simulink model "Telecontrol"  (R2024b)
settings: Solver=ode5  StartTime=0.0  StopTime=inf  FixedStep=1/600  RelTol=1e-3
undefined symbols (not defined in the file): Low
libraries: arduinolib x42, dspswit3 x12, etargetslib x10, simulink x6, canmsglib x6, svdutilitieslib x1
settings Model: SimulationMode=external  Creator=alexx  LastModifiedBy=Marwa
settings SolverCC: AutoInsertRateTranBlk=on
settings OptimizationCC: EnhancedBackFolding=on  PassReuseOutputArgsAs=Individual arguments  ZeroExternalMemoryAtStartup=off  ZeroInternalMemoryAtStartup=off  MaxStackSize=64  OptimizeBlockOrder=speed  DifferentSizesBufferReuse=on  OptimizationCustomize=off  EfficientTunableParamExpr=on
settings DebuggingCC: ParameterTunabilityLossMsg=error
settings HardwareCC: ProdBitPerPointer=32  ProdBitPerSizeT=32  ProdBitPerPtrDiffT=32  ProdLargestAtomicInteger=Long  ProdLargestAtomicFloat=Double  ProdWordSize=32  ProdHWDeviceType=ARM Compatible->ARM Cortex  UseEmbeddedCoderFeatures=off
settings SFSimCC: MATLABDynamicMemAlloc=off
settings RTWCC: Description=Embedded Coder  SystemTargetFile=ert.tlc  HardwareBoard=Arduino MKR WiFi 1010  TemplateMakefile=ert_default_tmf  Toolchain=Arduino ARM  BuildConfiguration=Faster Runs  GPUComputeCapability=3.5
settings CodeAppCC: ForceParamTrailComments=on  IgnoreCustomStorageClasses=off  OperatorAnnotations=on  SimulinkDataObjDesc=on  SFDataObjDesc=on  InsertBlockDesc=on
settings ERTTargetCC: SupportContinuousTime=on  SupportNonInlinedSFcns=on  SupportVariableSizeSignals=on  ExtModeTransport=3  ExtModeStaticAlloc=on  ExtModeAutomaticAllocSize=off  ExtModeStaticAllocSize=8192  ExtModeMexFile=ext_xcp  ExtModeIntrfLevel=Level2 - Open  InlinedParameterPlacement=Hierarchical  DynamicArrayContainerType=coder::array

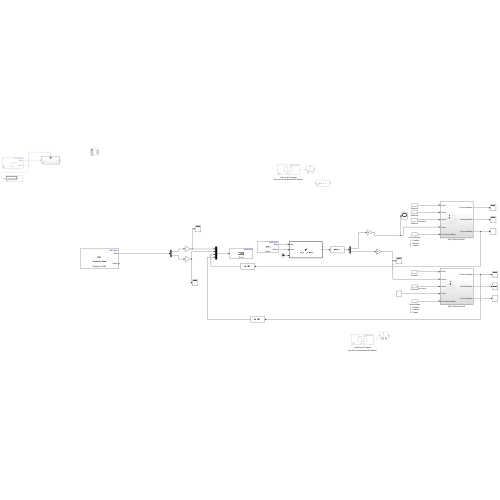
[thumbnail: Simulink's stored preview of the top-level diagram]
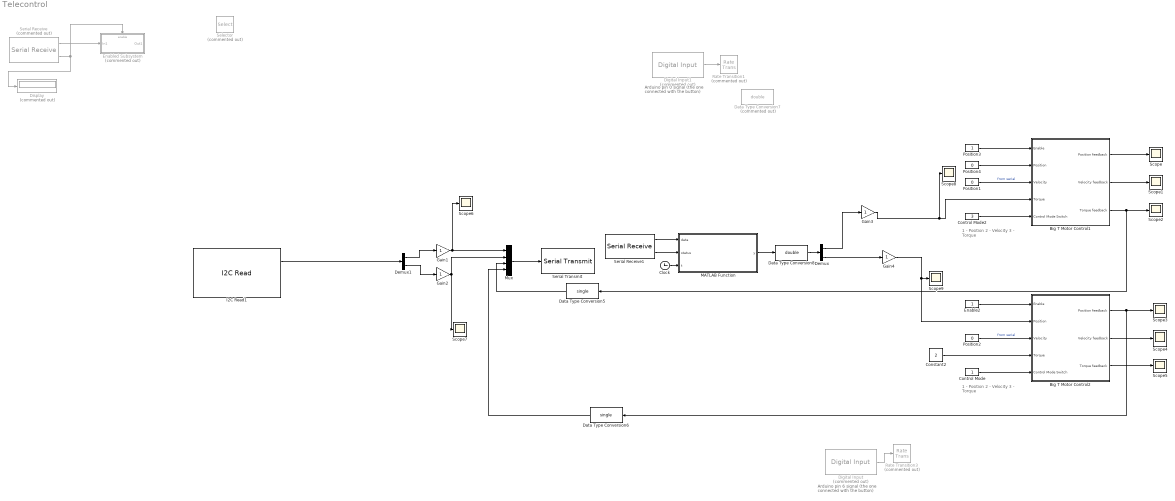
== system Telecontrol ==
  note: 1 - Position
      | 2 - Velocity
      | 3 - Torque
  note: Arduino pin 6 signal
      | (the one connected with the button)
  note: Arduino pin 0 signal
      | (the one connected with the button)
  note: 1 - Position
      | 2 - Velocity
      | 3 - Torque
  Big T Motor Control1 : Subsystem
  Big T Motor Control2 : Subsystem
  Clock : Clock
  Constant2 : Constant  Value=2
  Control Mode : Constant
  Control Mode2 : Constant  Value=3
  Data Type Conversion5 : DataTypeConversion  OutDataTypeStr=single  SaturateOnIntegerOverflow=off  RndMeth=Floor
  Data Type Conversion6 : DataTypeConversion  OutDataTypeStr=single  SaturateOnIntegerOverflow=off  RndMeth=Floor
  Data Type Conversion7 : DataTypeConversion  Commented=on  OutDataTypeStr=double  SaturateOnIntegerOverflow=off  RndMeth=Floor
  Data Type Conversion8 : DataTypeConversion  OutDataTypeStr=double  SaturateOnIntegerOverflow=off  RndMeth=Floor
  Demux : Demux  Outputs=2
  Demux1 : Demux  Outputs=2
  Digital Input : arduinolib/Digital Input  Commented=on  pinNumber=6  mode=Default  Direction=input  SampleTime=0.01  blockPlatform=arduino
      settings: SourceProductName=Common
  Digital Input1 : arduinolib/Digital Input  Commented=on  pinNumber=0  mode=Default  Direction=input  SampleTime=0.01  blockPlatform=arduino
      settings: SourceProductName=Common
  Display : Display  Commented=on
  Enable2 : Constant
  Enabled Subsystem : Subsystem  Commented=on  TreatAsAtomicUnit=on
  Gain{1..4} (4 alike) : Gain
  I2C Read1 : arduinolib/I2C Read  I2CModule=0  Mode=Master  SlaveAddress=45  SlaveByteOrder=LittleEndian  Direction=Receiver  RegisterAddressMode=off  RegisterAddress=0  SlaveDataType=single  DataLength=2  NoAck=off  RepeatedStart=off  OutputStatus=on  blockPlatform=ARDUINO  SampleTime=1/300
      settings: SourceProductName=Common
  MATLAB Function : MATLAB Function  TreatAsAtomicUnit=on
  Mux : Mux
  Position1 : Constant  Value=0
  Position2 : Constant  Value=0
  Position3 : Constant
  Position4 : Constant  Value=0
  Rate Transition1 : RateTransition  Commented=on  OutPortSampleTime=0.01
  Rate Transition3 : RateTransition  Commented=on  OutPortSampleTime=0.01
  Scope{,1..9} (10 alike) : Scope
  Selector : Selector  Commented=on  InputPortWidth=4  IndexOptions=Index vector (dialog)  Indices=[2 3]  OutputSizes=1
  Serial Receive : arduinolib/Serial Receive  Commented=on  portNumber=1  DataType=uint8  blockPlatform=ARDUINO  TimeOut=100  MaxDataLength=8  isARMArch=off  DataLengthOption=Length via dialog  Datalength=8  Header=[170.0]  Terminator=[187.0]  SampleTime=0.001  ShowOutStatus=on
      settings: SourceProductName=Common
  Serial Receive1 : arduinolib/Serial Receive  portNumber=0  DataType=single  blockPlatform=ARDUINO  TimeOut=0  MaxDataLength=10  isARMArch=off  DataLengthOption=Length via dialog  Datalength=2  Header=[170 85]  Terminator=[]  SampleTime=1/300  ShowOutStatus=on
      settings: SourceProductName=Common
  Serial Transmit : arduinolib/Serial Transmit  portNumber=0  sendmode=write  sendformat=Decimal  floatprecision=2  header=[170 85]  terminator=[]  blockPlatform=ARDUINO
      settings: SourceProductName=Common
  wires:
  Control Mode2/1 -> Big T Motor Control1/5(Control Mode Switch)
  Digital Input/1 -> Rate Transition3/1
  Position4/1 -> Big T Motor Control1/2(Position)
  Control Mode/1 -> Big T Motor Control2/5(Control Mode Switch)
  Big T Motor Control1/1(Position feedback) -> Scope/1
  Big T Motor Control1/2(Velocity feedback) -> Scope1/1
  Big T Motor Control1/3(Torque feedback) -> Data Type Conversion5/1, Scope2/1
  Big T Motor Control2/1(Position feedback) -> Data Type Conversion6/1, Scope3/1
  Big T Motor Control2/2(Velocity feedback) -> Scope4/1
  Big T Motor Control2/3(Torque feedback) -> Scope5/1
  Digital Input1/1 -> Rate Transition1/1
  Position1/1 -> Big T Motor Control1/3(Velocity)  "from serial"
  Constant2/1 -> Big T Motor Control2/4(Torque)
  Position2/1 -> Big T Motor Control2/3(Velocity)  "from serial"
  Serial Receive/2 -> Display/1, Enabled Subsystem/Enable
  Serial Receive/1 -> Enabled Subsystem/1(In1)
  Position3/1 -> Big T Motor Control1/1(Enable)
  Enable2/1 -> Big T Motor Control2/1(Enable)
  Serial Receive1/2 -> MATLAB Function/2(status)
  Mux/1 -> Serial Transmit/1
  Gain1/1 -> Mux/1, Scope6/1
  Gain2/1 -> Scope7/1, Mux/2
  Gain3/1 -> Scope8/1, Big T Motor Control1/4(Torque)
  Gain4/1 -> Big T Motor Control2/2(Position), Scope9/1
  Data Type Conversion8/1 -> Demux/1
  Demux/2 -> Gain4/1
  Demux/1 -> Gain3/1
  Data Type Conversion5/1 -> Mux/3
  Data Type Conversion6/1 -> Mux/4
  Serial Receive1/1 -> MATLAB Function/1(data)
  MATLAB Function/1(y) -> Data Type Conversion8/1
  Clock/1 -> MATLAB Function/3(t)
  I2C Read1/1 -> Demux1/1
  Demux1/1 -> Gain1/1
  Demux1/2 -> Gain2/1

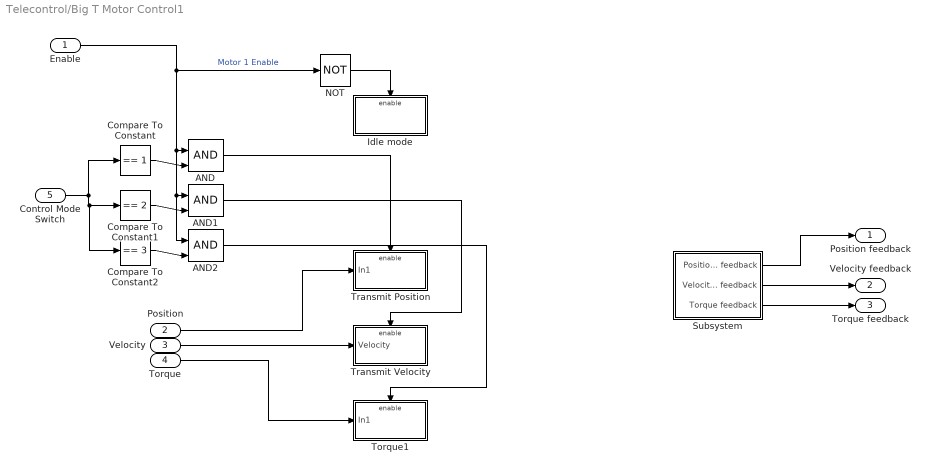
== system Telecontrol/Big T Motor Control1 ==
  Enable : Inport
  Position : Inport  Port=2  Unit=rad
  Velocity : Inport  Port=3  Unit=rad/s
  Torque : Inport  Port=4  Unit=N*m
  Control Mode Switch : Inport  Port=5
  AND : Logic  IconShape=distinctive  AllPortsSameDT=off  OutDataTypeStr=boolean
  AND1 : Logic  IconShape=distinctive  AllPortsSameDT=off  OutDataTypeStr=boolean
  AND2 : Logic  IconShape=distinctive  AllPortsSameDT=off  OutDataTypeStr=boolean
  Compare To Constant : simulink/Logic and Bit Operations/Compare To Constant  relop===  const=1  OutDataTypeStr=boolean
  Compare To Constant1 : simulink/Logic and Bit Operations/Compare To Constant  relop===  const=2  OutDataTypeStr=boolean
  Compare To Constant2 : simulink/Logic and Bit Operations/Compare To Constant  relop===  const=3  OutDataTypeStr=boolean
  Idle mode : Subsystem  TreatAsAtomicUnit=on
  NOT : Logic  Operator=NOT  AllPortsSameDT=off  OutDataTypeStr=boolean
  Subsystem : Subsystem
  Torque1 : Subsystem  TreatAsAtomicUnit=on
  Transmit Position : Subsystem  TreatAsAtomicUnit=on
  Transmit Velocity : Subsystem  TreatAsAtomicUnit=on
  Position feedback : Outport
  Velocity feedback : Outport  Port=2
  Torque feedback : Outport  Port=3
  wires:
  Position/1 -> Transmit Position/1(In1)
  Torque/1 -> Torque1/1(In1)
  Enable/1 -> AND2/1, AND1/1, AND/1, NOT/1  "Motor 1 Enable"
  NOT/1 -> Idle mode/Enable
  Control Mode Switch/1 -> Compare To Constant2/1, Compare To Constant1/1, Compare To Constant/1
  Velocity/1 -> Transmit Velocity/1(Velocity)
  Compare To Constant/1 -> AND/2
  AND/1 -> Transmit Position/Enable
  Compare To Constant1/1 -> AND1/2
  AND1/1 -> Transmit Velocity/Enable
  Compare To Constant2/1 -> AND2/2
  AND2/1 -> Torque1/Enable
  Subsystem/2(Velocity feedback) -> Velocity feedback/1
  Subsystem/1(Position feedback) -> Position feedback/1
  Subsystem/3(Torque feedback) -> Torque feedback/1

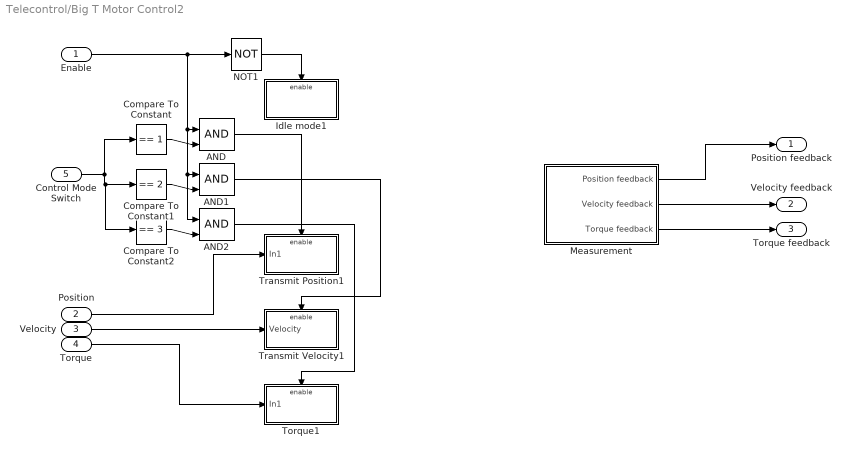
== system Telecontrol/Big T Motor Control2 ==
  Enable : Inport
  Position : Inport  Port=2  Unit=rad
  Velocity : Inport  Port=3  Unit=rad/s
  Torque : Inport  Port=4  Unit=N*m
  Control Mode Switch : Inport  Port=5
  AND : Logic  IconShape=distinctive  AllPortsSameDT=off  OutDataTypeStr=boolean
  AND1 : Logic  IconShape=distinctive  AllPortsSameDT=off  OutDataTypeStr=boolean
  AND2 : Logic  IconShape=distinctive  AllPortsSameDT=off  OutDataTypeStr=boolean
  Compare To Constant : simulink/Logic and Bit Operations/Compare To Constant  relop===  const=1  OutDataTypeStr=boolean
  Compare To Constant1 : simulink/Logic and Bit Operations/Compare To Constant  relop===  const=2  OutDataTypeStr=boolean
  Compare To Constant2 : simulink/Logic and Bit Operations/Compare To Constant  relop===  const=3  OutDataTypeStr=boolean
  Idle mode1 : Subsystem  TreatAsAtomicUnit=on
  Measurement : Subsystem
  NOT1 : Logic  Operator=NOT  AllPortsSameDT=off  OutDataTypeStr=boolean
  Torque1 : Subsystem  TreatAsAtomicUnit=on
  Transmit Position1 : Subsystem  TreatAsAtomicUnit=on
  Transmit Velocity1 : Subsystem  TreatAsAtomicUnit=on
  Position feedback : Outport
  Velocity feedback : Outport  Port=2
  Torque feedback : Outport  Port=3
  wires:
  Velocity/1 -> Transmit Velocity1/1(Velocity)
  Position/1 -> Transmit Position1/1(In1)
  Torque/1 -> Torque1/1(In1)
  NOT1/1 -> Idle mode1/Enable
  AND2/1 -> Torque1/Enable
  Control Mode Switch/1 -> Compare To Constant2/1, Compare To Constant1/1, Compare To Constant/1
  Compare To Constant1/1 -> AND1/2
  AND1/1 -> Transmit Velocity1/Enable
  Compare To Constant/1 -> AND/2
  Compare To Constant2/1 -> AND2/2
  AND/1 -> Transmit Position1/Enable
  Enable/1 -> NOT1/1, AND/1, AND2/1, AND1/1
  Measurement/1(Position feedback) -> Position feedback/1
  Measurement/2(Velocity feedback) -> Velocity feedback/1
  Measurement/3(Torque feedback) -> Torque feedback/1

== system Telecontrol/Enabled Subsystem ==
  In1 : Inport
  Enable : EnablePort
  Byte Unpack : svdutilitieslib/Byte Unpack  dimensions={[2]}  datatypes={'single'}  byteAlign=1  blockPlatform=arduinoert
  Out1 : Outport
  wires:
  In1/1 -> Byte Unpack/1
  Byte Unpack/1 -> Out1/1

== system Telecontrol/Big T Motor Control1/Idle mode ==
  Enable : EnablePort
  CAN Transmit1 : arduinolib/CAN Transmit  inputDataType=Raw data  BlockingMode_=off  BlockTimeout_=1  outputStatus=off  identifierType=Extended (29-bit identifier)  messageId=2097192  msgLength=0  remoteFrame=off
      settings: SourceProductName=Common

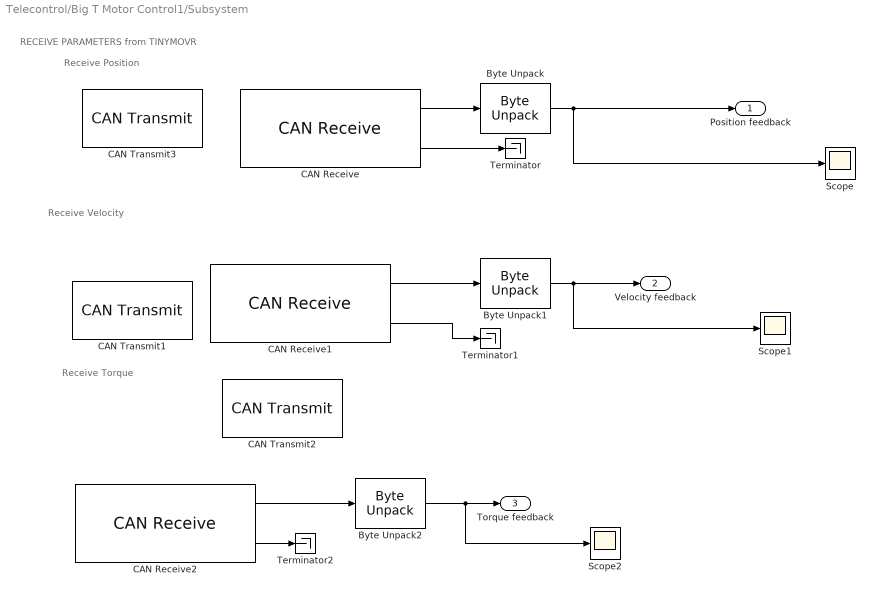
== system Telecontrol/Big T Motor Control1/Subsystem ==
  note: Receive Torque
  note: Receive Velocity
  note: Receive Position
  note: RECEIVE PARAMETERS from TINYMOVR
  Byte Unpack : etargetslib/Byte Unpack  dimensions={[1]}  datatypes={'single'}  byteAlign=1
  Byte Unpack1 : etargetslib/Byte Unpack  dimensions={[1]}  datatypes={'single'}  byteAlign=1
  Byte Unpack2 : etargetslib/Byte Unpack  dimensions={[1]}  datatypes={'single'}  byteAlign=1
  CAN Receive : arduinolib/CAN Receive  outputDataType=Raw data  identifierType=Extended (29-bit identifier)  messageId=2097207  msgLength=4  SampleTime=1/100  outputError=off  outputRemote=off
      settings: SourceProductName=Common
  CAN Receive1 : arduinolib/CAN Receive  outputDataType=Raw data  identifierType=Extended (29-bit identifier)  messageId=2097208  msgLength=4  SampleTime=1/100  outputError=off  outputRemote=off
      settings: SourceProductName=Common
  CAN Receive2 : arduinolib/CAN Receive  outputDataType=Raw data  identifierType=Extended (29-bit identifier)  messageId=2097185  msgLength=4  SampleTime=-1  outputError=off  outputRemote=off
      settings: SourceProductName=Common
  CAN Transmit1 : arduinolib/CAN Transmit  inputDataType=Raw data  BlockingMode_=off  BlockTimeout_=1  outputStatus=off  identifierType=Extended (29-bit identifier)  messageId=2097208  msgLength=0  remoteFrame=on
      settings: SourceProductName=Common
  CAN Transmit2 : arduinolib/CAN Transmit  inputDataType=Raw data  BlockingMode_=off  BlockTimeout_=1  outputStatus=off  identifierType=Extended (29-bit identifier)  messageId=2097185  msgLength=0  remoteFrame=on
      settings: SourceProductName=Common
  CAN Transmit3 : arduinolib/CAN Transmit  inputDataType=Raw data  BlockingMode_=off  BlockTimeout_=1  outputStatus=off  identifierType=Extended (29-bit identifier)  messageId=2097207  msgLength=0  remoteFrame=on
      settings: SourceProductName=Common
  Scope : Scope
  Scope1 : Scope
  Scope2 : Scope
  Terminator : Terminator
  Terminator1 : Terminator
  Terminator2 : Terminator
  Position feedback : Outport
  Velocity feedback : Outport  Port=2
  Torque feedback : Outport  Port=3
  wires:
  CAN Receive1/2 -> Terminator1/1
  Byte Unpack/1 -> Position feedback/1, Scope/1
  CAN Receive/1 -> Byte Unpack/1
  CAN Receive2/1 -> Byte Unpack2/1
  Byte Unpack2/1 -> Torque feedback/1, Scope2/1
  CAN Receive1/1 -> Byte Unpack1/1
  CAN Receive/2 -> Terminator/1
  Byte Unpack1/1 -> Velocity feedback/1, Scope1/1
  CAN Receive2/2 -> Terminator2/1

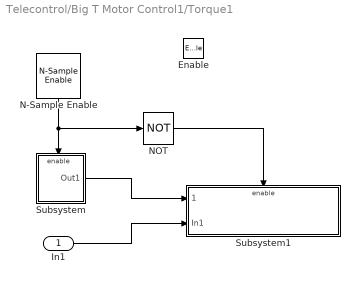
== system Telecontrol/Big T Motor Control1/Torque1 ==
  In1 : Inport
  Enable : EnablePort
  N-Sample Enable : dspswit3/N-Sample Enable  N=5  ActiveLevel=Low (0)  reset=off  TriggerType=Rising edge  Ts=1/100  DataType=Logical
  NOT : Logic  Operator=NOT  IconShape=distinctive  AllPortsSameDT=off  OutDataTypeStr=boolean
  Subsystem : Subsystem
  Subsystem1 : Subsystem
  wires:
  N-Sample Enable/1 -> Subsystem/Enable, NOT/1
  Subsystem/1(Out1) -> Subsystem1/1(" ")
  In1/1 -> Subsystem1/2(In1)
  NOT/1 -> Subsystem1/Enable

== system Telecontrol/Big T Motor Control1/Transmit Position ==
  In1 : Inport
  Enable : EnablePort
  N-Sample Enable : dspswit3/N-Sample Enable  N=5  ActiveLevel=Low (0)  reset=off  TriggerType=Rising edge  Ts=1/100  DataType=Logical
  NOT : Logic  Operator=NOT  IconShape=distinctive  AllPortsSameDT=off  OutDataTypeStr=boolean
  Subsystem : Subsystem
  Subsystem1 : Subsystem
  wires:
  N-Sample Enable/1 -> Subsystem/Enable, NOT/1
  Subsystem/1(Out1) -> Subsystem1/1(" ")
  In1/1 -> Subsystem1/2(In1)
  NOT/1 -> Subsystem1/Enable

== system Telecontrol/Big T Motor Control1/Transmit Velocity ==
  Velocity : Inport
  Enable : EnablePort
  N-Sample Enable : dspswit3/N-Sample Enable  N=5  ActiveLevel=Low (0)  reset=off  TriggerType=Rising edge  Ts=1/100  DataType=Logical
  NOT : Logic  Operator=NOT  IconShape=distinctive  AllPortsSameDT=off  OutDataTypeStr=boolean
  Subsystem : Subsystem
  Subsystem1 : Subsystem
  wires:
  N-Sample Enable/1 -> Subsystem/Enable, NOT/1
  Velocity/1 -> Subsystem1/1(Velocity)
  NOT/1 -> Subsystem1/Enable

== system Telecontrol/Big T Motor Control2/Idle mode1 ==
  Enable : EnablePort
  CAN Transmit1 : arduinolib/CAN Transmit  inputDataType=Raw data  BlockingMode_=off  BlockTimeout_=1  outputStatus=off  identifierType=Extended (29-bit identifier)  messageId=4194344  msgLength=0  remoteFrame=off
      settings: SourceProductName=Common

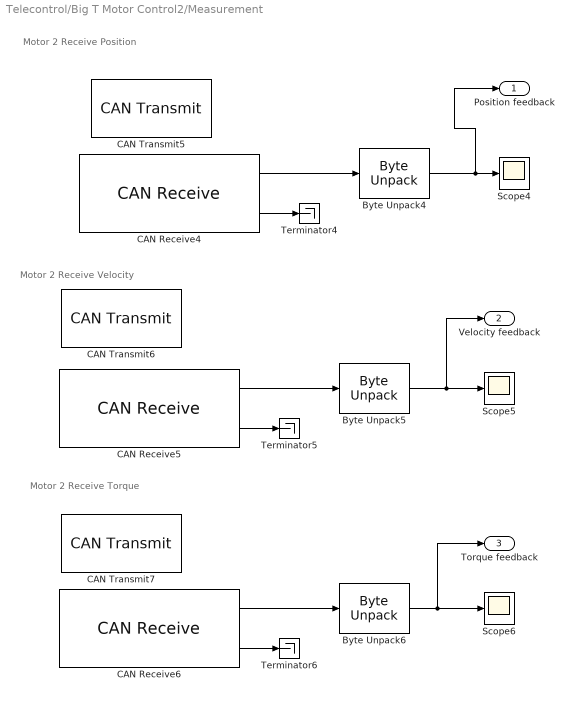
== system Telecontrol/Big T Motor Control2/Measurement ==
  note: Motor 2 Receive Torque
  note: Motor 2 Receive Velocity
  note: Motor 2 Receive Position
  Byte Unpack4 : etargetslib/Byte Unpack  dimensions={[1]}  datatypes={'single'}  byteAlign=1
  Byte Unpack5 : etargetslib/Byte Unpack  dimensions={[1]}  datatypes={'single'}  byteAlign=1
  Byte Unpack6 : etargetslib/Byte Unpack  dimensions={[1]}  datatypes={'single'}  byteAlign=1
  CAN Receive4 : arduinolib/CAN Receive  outputDataType=Raw data  identifierType=Extended (29-bit identifier)  messageId=4194359  msgLength=4  SampleTime=0.01  outputError=off  outputRemote=off
      settings: SourceProductName=Common
  CAN Receive5 : arduinolib/CAN Receive  outputDataType=Raw data  identifierType=Extended (29-bit identifier)  messageId=4194360  msgLength=4  SampleTime=0.01  outputError=off  outputRemote=off
      settings: SourceProductName=Common
  CAN Receive6 : arduinolib/CAN Receive  outputDataType=Raw data  identifierType=Extended (29-bit identifier)  messageId=4194337  msgLength=4  SampleTime=0.01  outputError=off  outputRemote=off
      settings: SourceProductName=Common
  CAN Transmit5 : arduinolib/CAN Transmit  inputDataType=Raw data  BlockingMode_=off  BlockTimeout_=1  outputStatus=off  identifierType=Extended (29-bit identifier)  messageId=4194359  msgLength=0  remoteFrame=on
      settings: SourceProductName=Common
  CAN Transmit6 : arduinolib/CAN Transmit  inputDataType=Raw data  BlockingMode_=off  BlockTimeout_=1  outputStatus=off  identifierType=Extended (29-bit identifier)  messageId=4194360  msgLength=0  remoteFrame=on
      settings: SourceProductName=Common
  CAN Transmit7 : arduinolib/CAN Transmit  inputDataType=Raw data  BlockingMode_=off  BlockTimeout_=1  outputStatus=off  identifierType=Extended (29-bit identifier)  messageId=4194337  msgLength=0  remoteFrame=on
      settings: SourceProductName=Common
  Scope4 : Scope
  Scope5 : Scope
  Scope6 : Scope
  Terminator4 : Terminator
  Terminator5 : Terminator
  Terminator6 : Terminator
  Position feedback : Outport
  Velocity feedback : Outport  Port=2
  Torque feedback : Outport  Port=3
  wires:
  CAN Receive5/1 -> Byte Unpack5/1
  CAN Receive4/1 -> Byte Unpack4/1
  Byte Unpack4/1 -> Position feedback/1, Scope4/1
  CAN Receive6/2 -> Terminator6/1
  CAN Receive6/1 -> Byte Unpack6/1
  Byte Unpack5/1 -> Velocity feedback/1, Scope5/1
  CAN Receive5/2 -> Terminator5/1
  CAN Receive4/2 -> Terminator4/1
  Byte Unpack6/1 -> Torque feedback/1, Scope6/1

== system Telecontrol/Big T Motor Control2/Torque1 ==
  In1 : Inport
  Enable : EnablePort
  N-Sample Enable : dspswit3/N-Sample Enable  N=5  ActiveLevel=Low (0)  reset=off  TriggerType=Rising edge  Ts=1/100  DataType=Logical
  NOT : Logic  Operator=NOT  IconShape=distinctive  AllPortsSameDT=off  OutDataTypeStr=boolean
  Subsystem : Subsystem
  Subsystem1 : Subsystem
  wires:
  N-Sample Enable/1 -> Subsystem/Enable, NOT/1
  Subsystem/1(Out1) -> Subsystem1/1(" ")
  In1/1 -> Subsystem1/2(In1)
  NOT/1 -> Subsystem1/Enable

== system Telecontrol/Big T Motor Control2/Transmit Position1 ==
  In1 : Inport
  Enable : EnablePort
  N-Sample Enable : dspswit3/N-Sample Enable  N=5  ActiveLevel=Low (0)  reset=off  TriggerType=Rising edge  Ts=1/100  DataType=Logical
  NOT : Logic  Operator=NOT  IconShape=distinctive  AllPortsSameDT=off  OutDataTypeStr=boolean
  Subsystem : Subsystem
  Subsystem1 : Subsystem
  wires:
  N-Sample Enable/1 -> Subsystem/Enable, NOT/1
  Subsystem/1(Out1) -> Subsystem1/1(" ")
  In1/1 -> Subsystem1/2(In1)
  NOT/1 -> Subsystem1/Enable

== system Telecontrol/Big T Motor Control2/Transmit Velocity1 ==
  Velocity : Inport
  Enable : EnablePort
  N-Sample Enable : dspswit3/N-Sample Enable  N=5  ActiveLevel=Low (0)  reset=off  TriggerType=Rising edge  Ts=1/100  DataType=Logical
  NOT : Logic  Operator=NOT  IconShape=distinctive  AllPortsSameDT=off  OutDataTypeStr=boolean
  Subsystem : Subsystem
  Subsystem1 : Subsystem
  wires:
  N-Sample Enable/1 -> Subsystem/Enable, NOT/1
  Velocity/1 -> Subsystem1/1(Velocity)
  NOT/1 -> Subsystem1/Enable

== system Telecontrol/Big T Motor Control1/Torque1/Subsystem ==
  Enable : EnablePort
  Byte Unpack : etargetslib/Byte Unpack  dimensions={[1]}  datatypes={'single'}  byteAlign=1
  CAN Receive : arduinolib/CAN Receive  outputDataType=Raw data  identifierType=Extended (29-bit identifier)  messageId=2097185  msgLength=4  SampleTime=1/100  outputError=off  outputRemote=off
      settings: SourceProductName=Common
  CAN Transmit3 : arduinolib/CAN Transmit  inputDataType=Raw data  BlockingMode_=off  BlockTimeout_=1  outputStatus=off  identifierType=Extended (29-bit identifier)  messageId=2097185  msgLength=0  remoteFrame=on
      settings: SourceProductName=Common
  Terminator : Terminator
  Out1 : Outport
  wires:
  CAN Receive/2 -> Terminator/1
  CAN Receive/1 -> Byte Unpack/1
  Byte Unpack/1 -> Out1/1

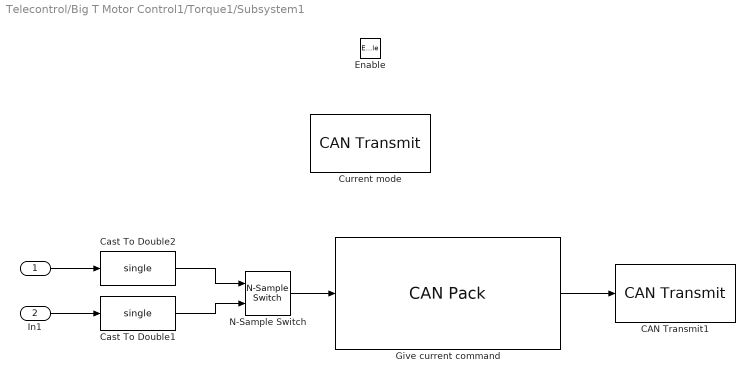
== system Telecontrol/Big T Motor Control1/Torque1/Subsystem1 ==
  " " : Inport
  In1 : Inport  Port=2
  Enable : EnablePort
  CAN Transmit1 : arduinolib/CAN Transmit  inputDataType=CAN Msg  BlockingMode_=off  BlockTimeout_=1  outputStatus=off  identifierType=Extended (29-bit identifier)  messageId=position_setpoint  msgLength=4  remoteFrame=off
      settings: SourceProductName=Common
  Cast To Double1 : DataTypeConversion  OutDataTypeStr=single  SaturateOnIntegerOverflow=off  RndMeth=Floor
  Cast To Double2 : DataTypeConversion  OutDataTypeStr=single  SaturateOnIntegerOverflow=off  RndMeth=Floor
  Current mode : arduinolib/CAN Transmit  inputDataType=Raw data  BlockingMode_=off  BlockTimeout_=1  outputStatus=off  identifierType=Extended (29-bit identifier)  messageId=2097195  msgLength=0  remoteFrame=off
      settings: SourceProductName=Common
  Give current command : canmsglib/CAN Pack  MsgList=(none)  MsgName=CAN Msg  MsgIDType=Extended (29-bit identifier)  MsgIdentifier=2097182  CANIDInput=off  MsgLength=4  Remote=off  ApplyMinMax=off  BusOutput=on  SignalInfo={ 'position', '0', '32', 'LE', 'single', 'Standard', '0', '1', '0', '-Inf', 'Inf' }
      settings: DataFormat=manually specified signals
  N-Sample Switch : dspswit3/N-Sample Switch  N=5  reset=off  TriggerType=Rising edge  Ts=1/100
  wires:
  Give current command/1 -> CAN Transmit1/1
  N-Sample Switch/1 -> Give current command/1
  Cast To Double1/1 -> N-Sample Switch/2
  " "/1 -> Cast To Double2/1
  In1/1 -> Cast To Double1/1
  Cast To Double2/1 -> N-Sample Switch/1

== system Telecontrol/Big T Motor Control1/Transmit Position/Subsystem ==
  Enable : EnablePort
  Byte Unpack : etargetslib/Byte Unpack  dimensions={[1]}  datatypes={'single'}  byteAlign=1
  CAN Receive : arduinolib/CAN Receive  outputDataType=Raw data  identifierType=Extended (29-bit identifier)  messageId=2097207  msgLength=4  SampleTime=1/100  outputError=off  outputRemote=off
      settings: SourceProductName=Common
  CAN Transmit3 : arduinolib/CAN Transmit  inputDataType=Raw data  BlockingMode_=off  BlockTimeout_=1  outputStatus=off  identifierType=Extended (29-bit identifier)  messageId=2097207  msgLength=0  remoteFrame=on
      settings: SourceProductName=Common
  Terminator : Terminator
  Out1 : Outport
  wires:
  CAN Receive/2 -> Terminator/1
  CAN Receive/1 -> Byte Unpack/1
  Byte Unpack/1 -> Out1/1

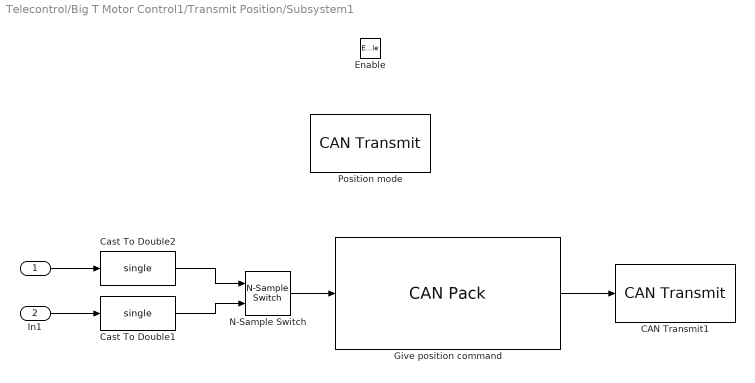
== system Telecontrol/Big T Motor Control1/Transmit Position/Subsystem1 ==
  " " : Inport
  In1 : Inport  Port=2
  Enable : EnablePort
  CAN Transmit1 : arduinolib/CAN Transmit  inputDataType=CAN Msg  BlockingMode_=off  BlockTimeout_=1  outputStatus=off  identifierType=Extended (29-bit identifier)  messageId=position_setpoint  msgLength=4  remoteFrame=off
      settings: SourceProductName=Common
  Cast To Double1 : DataTypeConversion  OutDataTypeStr=single  SaturateOnIntegerOverflow=off  RndMeth=Floor
  Cast To Double2 : DataTypeConversion  OutDataTypeStr=single  SaturateOnIntegerOverflow=off  RndMeth=Floor
  Give position command : canmsglib/CAN Pack  MsgList=(none)  MsgName=CAN Msg  MsgIDType=Extended (29-bit identifier)  MsgIdentifier=2097174  CANIDInput=off  MsgLength=4  Remote=off  ApplyMinMax=off  BusOutput=on  SignalInfo={ 'position', '0', '32', 'LE', 'single', 'Standard', '0', '1', '0', '-Inf', 'Inf' }
      settings: DataFormat=manually specified signals
  N-Sample Switch : dspswit3/N-Sample Switch  N=5  reset=off  TriggerType=Rising edge  Ts=1/100
  Position mode : arduinolib/CAN Transmit  inputDataType=Raw data  BlockingMode_=off  BlockTimeout_=1  outputStatus=off  identifierType=Extended (29-bit identifier)  messageId=2097193  msgLength=0  remoteFrame=off
      settings: SourceProductName=Common
  wires:
  Give position command/1 -> CAN Transmit1/1
  N-Sample Switch/1 -> Give position command/1
  Cast To Double1/1 -> N-Sample Switch/2
  " "/1 -> Cast To Double2/1
  In1/1 -> Cast To Double1/1
  Cast To Double2/1 -> N-Sample Switch/1

== system Telecontrol/Big T Motor Control1/Transmit Velocity/Subsystem ==
  Enable : EnablePort
  Velocity mode : arduinolib/CAN Transmit  inputDataType=Raw data  BlockingMode_=off  BlockTimeout_=1  outputStatus=off  identifierType=Extended (29-bit identifier)  messageId=2097194  msgLength=0  remoteFrame=off
      settings: SourceProductName=Common

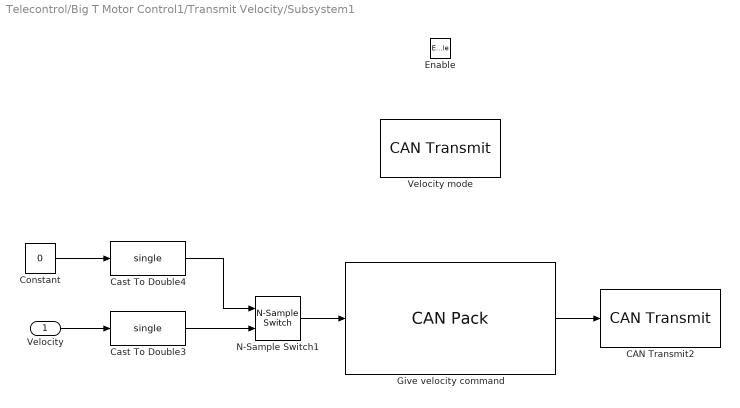
== system Telecontrol/Big T Motor Control1/Transmit Velocity/Subsystem1 ==
  Velocity : Inport  Unit=rad/s
  Enable : EnablePort
  CAN Transmit2 : arduinolib/CAN Transmit  inputDataType=CAN Msg  BlockingMode_=off  BlockTimeout_=1  outputStatus=off  identifierType=Extended (29-bit identifier)  messageId=2097173  msgLength=0  remoteFrame=off
      settings: SourceProductName=Common
  Cast To Double3 : DataTypeConversion  OutDataTypeStr=single  SaturateOnIntegerOverflow=off  RndMeth=Floor
  Cast To Double4 : DataTypeConversion  OutDataTypeStr=single  SaturateOnIntegerOverflow=off  RndMeth=Floor
  Constant : Constant  Value=0
  Give velocity command : canmsglib/CAN Pack  MsgList=(none)  MsgName=CAN Msg  MsgIDType=Extended (29-bit identifier)  MsgIdentifier=2097176  CANIDInput=off  MsgLength=4  Remote=off  ApplyMinMax=off  BusOutput=on  SignalInfo={ 'velocity', '0', '32', 'LE', 'single', 'Standard', '0', '1', '0', '-Inf', 'Inf' }
      settings: DataFormat=manually specified signals
  N-Sample Switch1 : dspswit3/N-Sample Switch  N=5  reset=off  TriggerType=Rising edge  Ts=1/100
  Velocity mode : arduinolib/CAN Transmit  inputDataType=Raw data  BlockingMode_=off  BlockTimeout_=1  outputStatus=off  identifierType=Extended (29-bit identifier)  messageId=2097194  msgLength=0  remoteFrame=off
      settings: SourceProductName=Common
  wires:
  Cast To Double4/1 -> N-Sample Switch1/1
  Velocity/1 -> Cast To Double3/1
  Constant/1 -> Cast To Double4/1
  N-Sample Switch1/1 -> Give velocity command/1
  Cast To Double3/1 -> N-Sample Switch1/2
  Give velocity command/1 -> CAN Transmit2/1

== system Telecontrol/Big T Motor Control2/Torque1/Subsystem ==
  Enable : EnablePort
  Byte Unpack : etargetslib/Byte Unpack  dimensions={[1]}  datatypes={'single'}  byteAlign=1
  CAN Receive : arduinolib/CAN Receive  outputDataType=Raw data  identifierType=Extended (29-bit identifier)  messageId=4194337  msgLength=4  SampleTime=1/100  outputError=off  outputRemote=off
      settings: SourceProductName=Common
  CAN Transmit3 : arduinolib/CAN Transmit  inputDataType=Raw data  BlockingMode_=off  BlockTimeout_=1  outputStatus=off  identifierType=Extended (29-bit identifier)  messageId=4194337  msgLength=0  remoteFrame=on
      settings: SourceProductName=Common
  Terminator : Terminator
  Out1 : Outport
  wires:
  CAN Receive/2 -> Terminator/1
  CAN Receive/1 -> Byte Unpack/1
  Byte Unpack/1 -> Out1/1

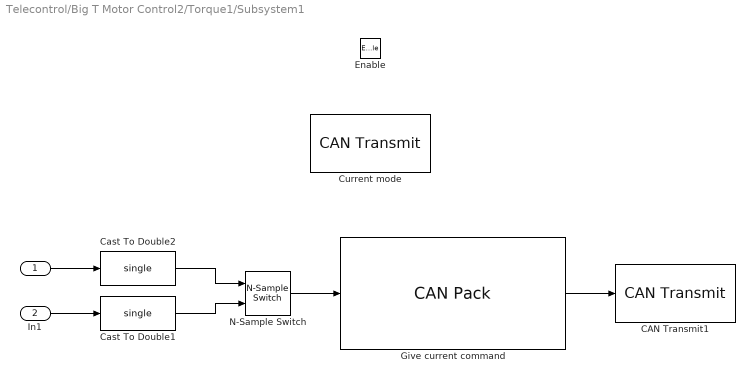
== system Telecontrol/Big T Motor Control2/Torque1/Subsystem1 ==
  " " : Inport
  In1 : Inport  Port=2
  Enable : EnablePort
  CAN Transmit1 : arduinolib/CAN Transmit  inputDataType=CAN Msg  BlockingMode_=off  BlockTimeout_=1  outputStatus=off  identifierType=Extended (29-bit identifier)  messageId=position_setpoint  msgLength=4  remoteFrame=off
      settings: SourceProductName=Common
  Cast To Double1 : DataTypeConversion  OutDataTypeStr=single  SaturateOnIntegerOverflow=off  RndMeth=Floor
  Cast To Double2 : DataTypeConversion  OutDataTypeStr=single  SaturateOnIntegerOverflow=off  RndMeth=Floor
  Current mode : arduinolib/CAN Transmit  inputDataType=Raw data  BlockingMode_=off  BlockTimeout_=1  outputStatus=off  identifierType=Extended (29-bit identifier)  messageId=4194347  msgLength=0  remoteFrame=off
      settings: SourceProductName=Common
  Give current command : canmsglib/CAN Pack  MsgList=(none)  MsgName=CAN Msg  MsgIDType=Extended (29-bit identifier)  MsgIdentifier=4194334  CANIDInput=off  MsgLength=4  Remote=off  ApplyMinMax=off  BusOutput=on  SignalInfo={ 'position', '0', '32', 'LE', 'single', 'Standard', '0', '1', '0', '-Inf', 'Inf' }
      settings: DataFormat=manually specified signals
  N-Sample Switch : dspswit3/N-Sample Switch  N=5  reset=off  TriggerType=Rising edge  Ts=1/100
  wires:
  Give current command/1 -> CAN Transmit1/1
  N-Sample Switch/1 -> Give current command/1
  Cast To Double1/1 -> N-Sample Switch/2
  " "/1 -> Cast To Double2/1
  In1/1 -> Cast To Double1/1
  Cast To Double2/1 -> N-Sample Switch/1

== system Telecontrol/Big T Motor Control2/Transmit Position1/Subsystem ==
  Enable : EnablePort
  Byte Unpack : etargetslib/Byte Unpack  dimensions={[1]}  datatypes={'single'}  byteAlign=1
  CAN Receive : arduinolib/CAN Receive  outputDataType=Raw data  identifierType=Extended (29-bit identifier)  messageId=4194345  msgLength=4  SampleTime=1/100  outputError=off  outputRemote=off
      settings: SourceProductName=Common
  CAN Transmit3 : arduinolib/CAN Transmit  inputDataType=Raw data  BlockingMode_=off  BlockTimeout_=1  outputStatus=off  identifierType=Extended (29-bit identifier)  messageId=2097207  msgLength=0  remoteFrame=on
      settings: SourceProductName=Common
  Terminator : Terminator
  Out1 : Outport
  wires:
  CAN Receive/2 -> Terminator/1
  CAN Receive/1 -> Byte Unpack/1
  Byte Unpack/1 -> Out1/1

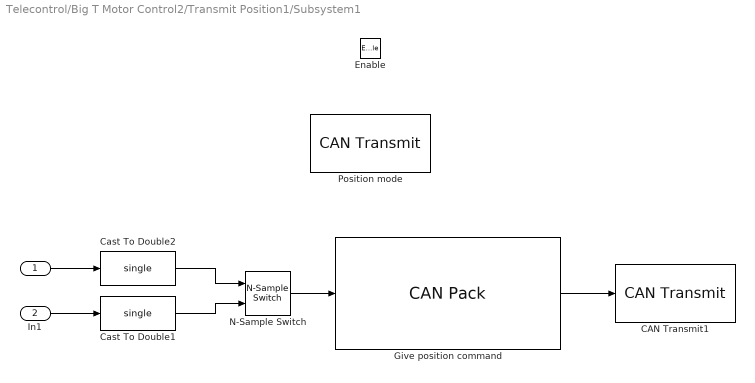
== system Telecontrol/Big T Motor Control2/Transmit Position1/Subsystem1 ==
  " " : Inport
  In1 : Inport  Port=2
  Enable : EnablePort
  CAN Transmit1 : arduinolib/CAN Transmit  inputDataType=CAN Msg  BlockingMode_=off  BlockTimeout_=1  outputStatus=off  identifierType=Extended (29-bit identifier)  messageId=position_setpoint  msgLength=4  remoteFrame=off
      settings: SourceProductName=Common
  Cast To Double1 : DataTypeConversion  OutDataTypeStr=single  SaturateOnIntegerOverflow=off  RndMeth=Floor
  Cast To Double2 : DataTypeConversion  OutDataTypeStr=single  SaturateOnIntegerOverflow=off  RndMeth=Floor
  Give position command : canmsglib/CAN Pack  MsgList=(none)  MsgName=CAN Msg  MsgIDType=Extended (29-bit identifier)  MsgIdentifier=4194326  CANIDInput=off  MsgLength=4  Remote=off  ApplyMinMax=off  BusOutput=on  SignalInfo={ 'position', '0', '32', 'LE', 'single', 'Standard', '0', '1', '0', '-Inf', 'Inf' }
      settings: DataFormat=manually specified signals
  N-Sample Switch : dspswit3/N-Sample Switch  N=5  reset=off  TriggerType=Rising edge  Ts=1/100
  Position mode : arduinolib/CAN Transmit  inputDataType=Raw data  BlockingMode_=off  BlockTimeout_=1  outputStatus=off  identifierType=Extended (29-bit identifier)  messageId=4194345  msgLength=0  remoteFrame=off
      settings: SourceProductName=Common
  wires:
  Give position command/1 -> CAN Transmit1/1
  N-Sample Switch/1 -> Give position command/1
  Cast To Double1/1 -> N-Sample Switch/2
  " "/1 -> Cast To Double2/1
  In1/1 -> Cast To Double1/1
  Cast To Double2/1 -> N-Sample Switch/1

== system Telecontrol/Big T Motor Control2/Transmit Velocity1/Subsystem ==
  Enable : EnablePort
  Velocity mode : arduinolib/CAN Transmit  inputDataType=Raw data  BlockingMode_=off  BlockTimeout_=1  outputStatus=off  identifierType=Extended (29-bit identifier)  messageId=4194346  msgLength=0  remoteFrame=off
      settings: SourceProductName=Common

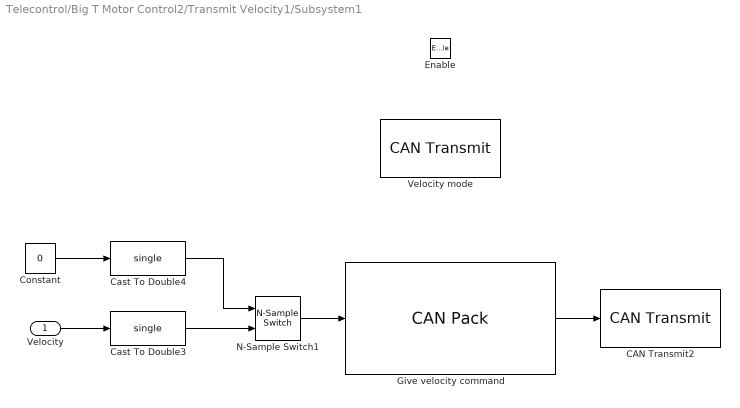
== system Telecontrol/Big T Motor Control2/Transmit Velocity1/Subsystem1 ==
  Velocity : Inport  Unit=rad/s
  Enable : EnablePort
  CAN Transmit2 : arduinolib/CAN Transmit  inputDataType=CAN Msg  BlockingMode_=off  BlockTimeout_=1  outputStatus=off  identifierType=Extended (29-bit identifier)  messageId=2097173  msgLength=0  remoteFrame=off
      settings: SourceProductName=Common
  Cast To Double3 : DataTypeConversion  OutDataTypeStr=single  SaturateOnIntegerOverflow=off  RndMeth=Floor
  Cast To Double4 : DataTypeConversion  OutDataTypeStr=single  SaturateOnIntegerOverflow=off  RndMeth=Floor
  Constant : Constant  Value=0
  Give velocity command : canmsglib/CAN Pack  MsgList=(none)  MsgName=CAN Msg  MsgIDType=Extended (29-bit identifier)  MsgIdentifier=4194328  CANIDInput=off  MsgLength=4  Remote=off  ApplyMinMax=off  BusOutput=on  SignalInfo={ 'velocity', '0', '32', 'LE', 'single', 'Standard', '0', '1', '0', '-Inf', 'Inf' }
      settings: DataFormat=manually specified signals
  N-Sample Switch1 : dspswit3/N-Sample Switch  N=5  reset=off  TriggerType=Rising edge  Ts=1/100
  Velocity mode : arduinolib/CAN Transmit  inputDataType=Raw data  BlockingMode_=off  BlockTimeout_=1  outputStatus=off  identifierType=Extended (29-bit identifier)  messageId=4194346  msgLength=0  remoteFrame=off
      settings: SourceProductName=Common
  wires:
  Cast To Double4/1 -> N-Sample Switch1/1
  Velocity/1 -> Cast To Double3/1
  Constant/1 -> Cast To Double4/1
  N-Sample Switch1/1 -> Give velocity command/1
  Cast To Double3/1 -> N-Sample Switch1/2
  Give velocity command/1 -> CAN Transmit2/1

== matlab function Telecontrol/MATLAB Function ==
  data: data input; y output; status input; t input
function y = hold_with_timeout(data, status, t)
%#codegen
persistent last_t last_y init
safe_value = [0.0;0.0];
timeout_s = 2;
if isempty(init)
    last_t = t;
    last_y = safe_value + zeros(size(data),'like',data);
    init = true;
end
if status==1
    last_y = data;
    last_t = t;
end
if (t - last_t) > timeout_s
    y = safe_value + zeros(size(data),'like',data);
else
    y = last_y;
end
